simulink model "pospoliy_4gdl_discretizzato"  (R2021a)
settings: Solver=VariableStepAuto  StartTime=0.0  StopTime=2  RelTol=1e-3
values from neighbouring files (symbols this model uses):
  my = config_dc(pary)    [mainy.m]
  pary = parametriy ()    [mainy.m]
  ppy_c = pos_poli_cc_y(my, ac, 2)    [mainy.m]
  ppy_m = pos_poli_cc_y(my, ac, 1)    [mainy.m]
undefined symbols (not defined in the file or in its folder): accelerazioniy, Evaluate_Trajectory
libraries: simulink x2
settings Model: Creator=stefa  LastModifiedBy=stefa

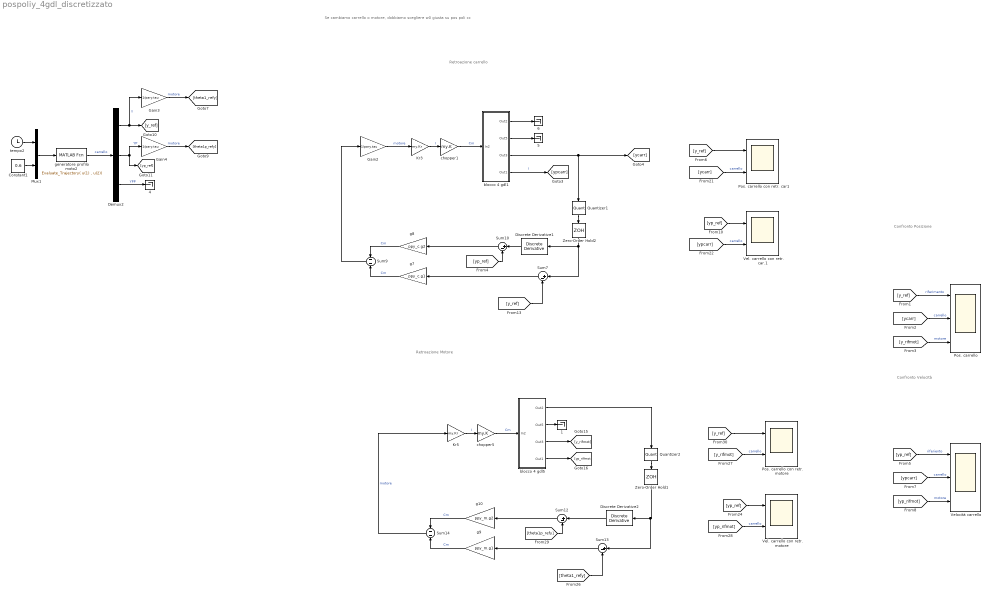
== system pospoliy_4gdl_discretizzato ==
  note: Retroazione carrello
  note: Se cambiamo carrello o motore, dobbiamo scegliere w0 giusta su pos poli cc
  note: Retroazione Motore
  note: Confronto Posizione
  note: Confronto
      | Velocità
   {1,4..6} (4 alike) : Terminator
  Constant1 : Constant  Value=0.6
  Demux2 : Demux  Outputs=3
  Discrete Derivative1 : simulink/Discrete/Discrete Derivative  gainval=1  ICPrevScaledInput=0.0  OutMin=[]  OutMax=[]  OutDataType=fixdt(1, 16)  OutScaling=2^-10  DoSatur=off
  Discrete Derivative2 : simulink/Discrete/Discrete Derivative  gainval=1.0  ICPrevScaledInput=0.0  OutMin=[]  OutMax=[]  OutDataType=fixdt(1, 16)  OutScaling=2^-10  DoSatur=off
  Gain2 : Gain  Gain=1/pary.tau
  Gain3 : Gain  Gain=1/pary.tau
  Gain4 : Gain  Gain=1/pary.tau
  Kr3 : Gain  Gain=my.Kr
  Kr5 : Gain  Gain=my.Kr
  Mux1 : Mux  Inputs=2
  "Pos. carrello " : Scope  NumInputPorts=3
  Pos. carrello con retr. car1 : Scope  NumInputPorts=2
  Pos. carrello con retr. motore : Scope  NumInputPorts=2
  Quantizer1 : Quantizer  QuantizationInterval=10/4096
  Quantizer2 : Quantizer  QuantizationInterval=10/4096
  Sum{7,10,12..13} (4 alike) : Sum  Inputs=|+-
  Sum14 : Sum  Inputs=--
  Sum9 : Sum  Inputs=--
  Vel. carrello con retr. car.1 : Scope  NumInputPorts=2
  Vel. carrello con retr. motore : Scope  NumInputPorts=2
  Velocità carrello : Scope  NumInputPorts=3
  Zero-Order Hold1 : ZeroOrderHold  SampleTime=0.001
  Zero-Order Hold2 : ZeroOrderHold  SampleTime=0.001
  blocco 4 gdl1 : Subsystem
  blocco 4 gdl5 : Subsystem
  chopper1 : Gain  Gain=my.K
  chopper5 : Gain  Gain=my.K
  g10 : Gain  Gain=ppy_m.g2
  g7 : Gain  Gain=ppy_c.g1
  g8 : Gain  Gain=ppy_c.g2
  g9 : Gain  Gain=ppy_m.g1
  generatore profilo moto2 : MATLABFcn  MATLABFcn=Evaluate_Trajectory( u(1) , u(2))  OutputDimensions=3
  tempo2 : Clock
  wires:
  chopper1/1 -> blocco 4 gdl1/1(In2)  "Cm"
  blocco 4 gdl1/3(Out3) -> [ycarr], Quantizer1/1
  Mux1/1 -> generatore profilo moto2/1
  Constant1/1 -> Mux1/2
  Demux2/2 -> Gain4/1, [yp_ref]  "YP"
  Kr3/1 -> chopper1/1  "I"
  generatore profilo moto2/1 -> Demux2/1  "carrello"
  Gain2/1 -> Kr3/1  "motore"
  Sum10/1 -> g8/1
  Demux2/3 -> " 4"/1  "YPP"
  Demux2/1 -> [y_ref], Gain3/1  "Y"
  [yp_ref] -> Vel. carrello con retr. car.1/1
  [yp_ref] -> Sum10/2
  g7/1 -> Sum9/2  "Cm"
  [ycarr] -> Pos. carrello con retr. car1/2  "carrello"
  [y_ref] -> Pos. carrello con retr. car1/1
  g8/1 -> Sum9/1  "Cm"
  [y_ref] -> Sum7/2
  Sum7/1 -> g7/1
  [yp_rifmot] -> Vel. carrello con retr. motore/2  "carrello"
  [ypcarr] -> Vel. carrello con retr. car.1/2  "carrello"
  Gain4/1 -> [theta1p_refy]  "motore"
  Kr5/1 -> chopper5/1  "I"
  Gain3/1 -> [theta1_refy]  "motore"
  blocco 4 gdl5/3(Out3) -> [y_rifmot]
  blocco 4 gdl5/4(Out1) -> [yp_rifmot]
  [theta1_refy] -> Sum13/2
  tempo2/1 -> Mux1/1
  [y_rifmot] -> Pos. carrello con retr. motore/2  "carrello"
  g10/1 -> Sum14/1  "Cm"
  blocco 4 gdl1/2(Out5) -> " 5"/1
  chopper5/1 -> blocco 4 gdl5/1(In2)  "Cm"
  [theta1p_refy] -> Sum12/2
  [y_ref] -> Pos. carrello con retr. motore/1
  [yp_ref] -> Vel. carrello con retr. motore/1
  g9/1 -> Sum14/2  "Cm"
  Sum12/1 -> g10/1
  Sum13/1 -> g9/1
  Sum14/1 -> Kr5/1  "motore"
  blocco 4 gdl1/1(Out2) -> " 6"/1
  [ypcarr] -> Velocità carrello/2  "carrello"
  [y_rifmot] -> "Pos. carrello "/3  "motore"
  [y_ref] -> "Pos. carrello "/1  "riferimento"
  [yp_rifmot] -> Velocità carrello/3  "motore"
  [yp_ref] -> Velocità carrello/1  "riferiento"
  Zero-Order Hold2/1 -> Discrete Derivative1/1, Sum7/1
  Discrete Derivative1/1 -> Sum10/1
  Quantizer1/1 -> Zero-Order Hold2/1
  Zero-Order Hold1/1 -> Sum13/1, Discrete Derivative2/1
  Quantizer2/1 -> Zero-Order Hold1/1
  blocco 4 gdl5/1(Out2) -> Quantizer2/1
  Discrete Derivative2/1 -> Sum12/1
  blocco 4 gdl5/2(Out5) -> " 1"/1
  [ycarr] -> "Pos. carrello "/2  "carrello"
  blocco 4 gdl1/4(Out1) -> [ypcarr]  "I"
  Sum9/1 -> Gain2/1

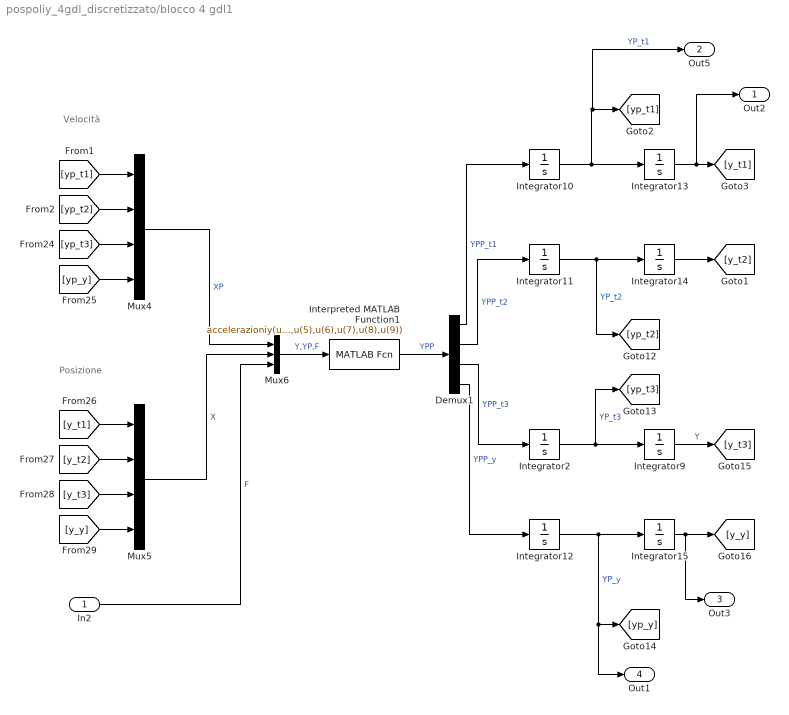
== system pospoliy_4gdl_discretizzato/blocco 4 gdl1 ==
  note: Posizione
  note: Velocità
  In2 : Inport
  Demux1 : Demux
  Integrator{2,9..15} (8 alike) : Integrator
  Interpreted MATLAB Function1 : MATLABFcn  MATLABFcn=accelerazioniy(u(1),u(2),u(3),u(4),u(5),u(6),u(7),u(8),u(9))  OutputDimensions=4
  Mux4 : Mux
  Mux5 : Mux
  Mux6 : Mux  Inputs=3
  Out2 : Outport
  Out5 : Outport  Port=2
  Out3 : Outport  Port=3
  Out1 : Outport  Port=4
  wires:
  Integrator15/1 -> Out3/1, [y_y]
  [yp_t2] -> Mux4/2
  [y_y] -> Mux5/4
  Demux1/2 -> Integrator11/1  "YPP_t2"
  Demux1/1 -> Integrator10/1  "YPP_t1"
  Mux6/1 -> Interpreted MATLAB Function1/1  "Y,YP,F"
  Demux1/3 -> Integrator2/1  "YPP_t3"
  Integrator2/1 -> [yp_t3], Integrator9/1  "YP_t3"
  Mux5/1 -> Mux6/2  "X"
  [y_t2] -> Mux5/2
  [y_t3] -> Mux5/3
  [yp_y] -> Mux4/4
  Integrator11/1 -> [yp_t2], Integrator14/1  "YP_t2"
  Integrator14/1 -> [y_t2]
  [yp_t3] -> Mux4/3
  In2/1 -> Mux6/3  "F"
  Integrator10/1 -> Out5/1, [yp_t1], Integrator13/1  "YP_t1"
  Demux1/4 -> Integrator12/1  "YPP_y"
  Mux4/1 -> Mux6/1  "XP"
  [yp_t1] -> Mux4/1
  [y_t1] -> Mux5/1
  Integrator9/1 -> [y_t3]  "Y"
  Integrator12/1 -> Out1/1, [yp_y], Integrator15/1  "YP_y"
  Integrator13/1 -> Out2/1, [y_t1]
  Interpreted MATLAB Function1/1 -> Demux1/1  "YPP"

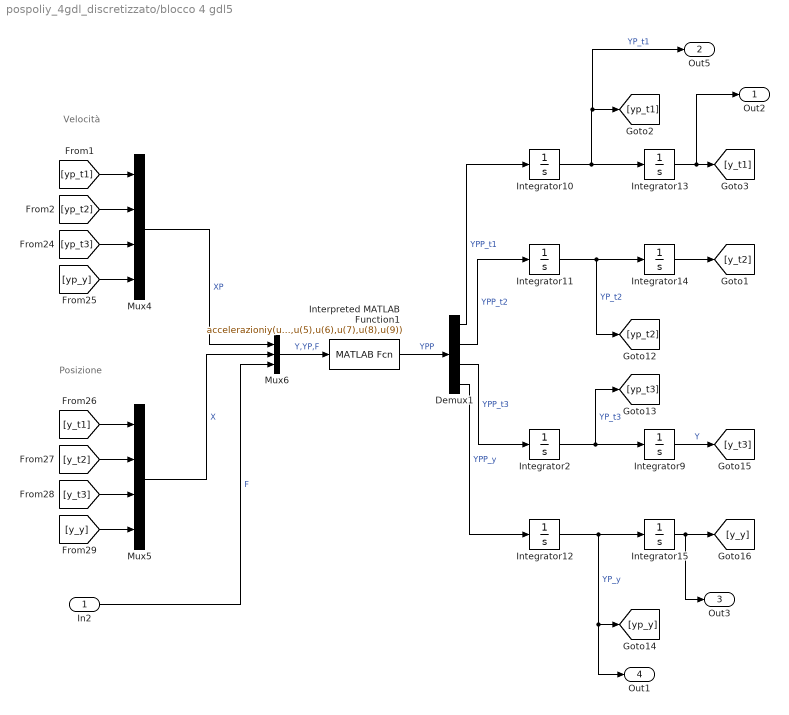
== system pospoliy_4gdl_discretizzato/blocco 4 gdl5 ==
  note: Posizione
  note: Velocità
  In2 : Inport
  Demux1 : Demux
  Integrator{2,9..15} (8 alike) : Integrator
  Interpreted MATLAB Function1 : MATLABFcn  MATLABFcn=accelerazioniy(u(1),u(2),u(3),u(4),u(5),u(6),u(7),u(8),u(9))  OutputDimensions=4
  Mux4 : Mux
  Mux5 : Mux
  Mux6 : Mux  Inputs=3
  Out2 : Outport
  Out5 : Outport  Port=2
  Out3 : Outport  Port=3
  Out1 : Outport  Port=4
  wires:
  Mux4/1 -> Mux6/1  "XP"
  Integrator9/1 -> [y_t3]  "Y"
  [y_t2] -> Mux5/2
  [yp_t1] -> Mux4/1
  Integrator13/1 -> Out2/1, [y_t1]
  Demux1/4 -> Integrator12/1  "YPP_y"
  Integrator12/1 -> Out1/1, [yp_y], Integrator15/1  "YP_y"
  [yp_t3] -> Mux4/3
  Integrator2/1 -> [yp_t3], Integrator9/1  "YP_t3"
  Integrator11/1 -> [yp_t2], Integrator14/1  "YP_t2"
  Demux1/1 -> Integrator10/1  "YPP_t1"
  Integrator10/1 -> Out5/1, [yp_t1], Integrator13/1  "YP_t1"
  [y_t1] -> Mux5/1
  Mux5/1 -> Mux6/2  "X"
  [y_t3] -> Mux5/3
  Demux1/2 -> Integrator11/1  "YPP_t2"
  Interpreted MATLAB Function1/1 -> Demux1/1  "YPP"
  [yp_t2] -> Mux4/2
  [yp_y] -> Mux4/4
  Integrator14/1 -> [y_t2]
  Integrator15/1 -> Out3/1, [y_y]
  Demux1/3 -> Integrator2/1  "YPP_t3"
  Mux6/1 -> Interpreted MATLAB Function1/1  "Y,YP,F"
  [y_y] -> Mux5/4
  In2/1 -> Mux6/3  "F"
